simulink subsystem "ADIS16460"  (R2021a)
settings: Solver=VariableStepAuto  StartTime=0.0  StopTime=10.0  RelTol=1e-3
undefined symbols (not defined in the file): acc, gyro, max_ref_temp, misalign
libraries: simulink x8, dspsrcs4 x6, dspmtrx3 x2
settings Model: Creator=jmher  LastModifiedBy=Laura

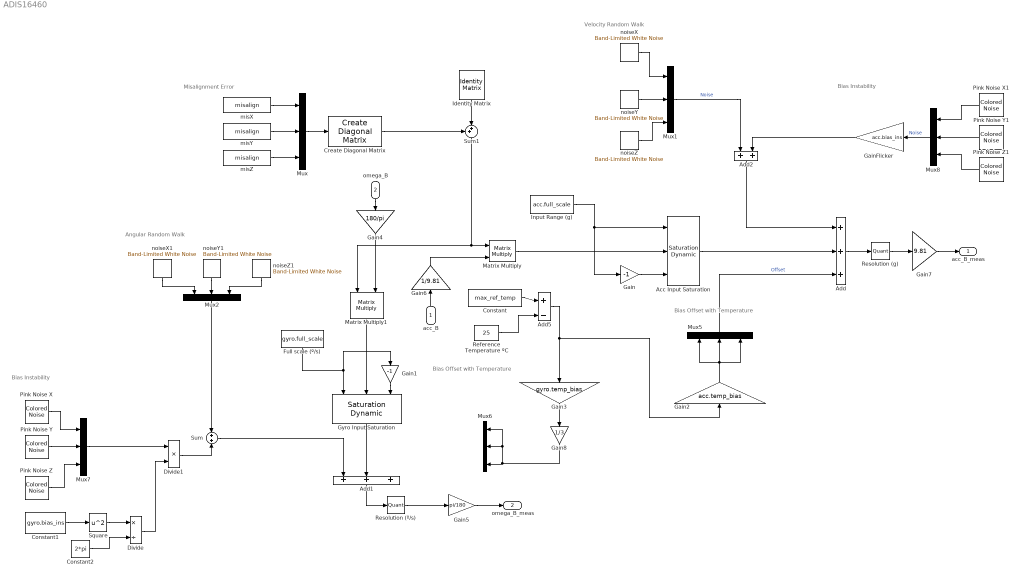
== system ADIS16460 ==
  note: Velocity Random Walk
  note: Bias Offset with Temperature
  note: Misalignment Error
  note: Bias Offset with Temperature
  note: Bias Instability
  note: Angular Random Walk
  note: Bias Instability
  acc_B : Inport  PortDimensions=3
  omega_B : Inport  Port=2  PortDimensions=3
  Acc Input Saturation : simulink/Discontinuities/Saturation Dynamic  OutMin=[]  OutMax=[]  OutDataTypeStr=Inherit: Same as second input  OutDataType=fixdt(1, 16)  OutScaling=2^-10  DoSatur=off
  Add : Sum  Inputs=+|+|+
  Add1 : Sum  Inputs=+|+|+
  Add2 : Sum  Inputs=+|+
  Add5 : Sum  Inputs=+|-
  Constant : Constant  Value=max_ref_temp
  Constant1 : Constant  Value=gyro.bias_ins
  Constant2 : Constant  Value=2*pi
  Create Diagonal Matrix : dspmtrx3/Create Diagonal Matrix
      settings: SourceProductBaseCode=DS
  Divide : Product  Inputs=*/
  Divide1 : Product  Inputs=**
  Full scale (º/s) : Constant  Value=gyro.full_scale
  Gain : Gain  Gain=-1
  Gain1 : Gain  Gain=-1
  Gain2 : Gain  Gain=acc.temp_bias
  Gain3 : Gain  Gain=gyro.temp_bias
  Gain4 : Gain  Gain=180/pi
  Gain5 : Gain  Gain=pi/180
  Gain6 : Gain  Gain=1/9.81
  Gain7 : Gain  Gain=9.81
  Gain8 : Gain  Gain=1/3
  GainFlicker : Gain  Gain=acc.bias_ins
  Gyro Input Saturation : simulink/Discontinuities/Saturation Dynamic  OutMin=[]  OutMax=[]  OutDataTypeStr=Inherit: Same as second input  OutDataType=fixdt(1, 16)  OutScaling=2^-10  DoSatur=off
  Identity Matrix : dspmtrx3/Identity Matrix  Inherit=off  N=3  Ts=1  dataType=double  isSigned=on  wordLen=16  udDataType=sfix(16)  fracBitsMode=Best precision  numFracBits=15  OutDataTypeStr=double  LastOutDataTypeStr=double
  Input Range (g) : Constant  Value=acc.full_scale
  Matrix Multiply : Product  Multiplication=Matrix(*)
  Matrix Multiply1 : Product  Multiplication=Matrix(*)
  Mux{,1..2,5..8} (7 alike) : Mux  Inputs=3
  Pink Noise X : dspsrcs4/Colored Noise  Color=pink  InverseFrequencyPower=biasAcc  BoundedOutput=off  NumChannels=1  OutputDataType=double  SamplesPerFrame=1  SampleTime=1/40  RandomStream=mt19937ar with seed  Seed=12237  SimulateUsing=Interpreted execution
      settings: SourceProductBaseCode=DS
  Pink Noise X1 : dspsrcs4/Colored Noise  Color=pink  InverseFrequencyPower=biasAcc  BoundedOutput=off  NumChannels=1  OutputDataType=double  SamplesPerFrame=1  SampleTime=1/40  RandomStream=mt19937ar with seed  Seed=6237342  SimulateUsing=Interpreted execution
      settings: SourceProductBaseCode=DS
  Pink Noise Y : dspsrcs4/Colored Noise  Color=pink  InverseFrequencyPower=biasAcc  BoundedOutput=off  NumChannels=1  OutputDataType=double  SamplesPerFrame=1  SampleTime=1/40  RandomStream=mt19937ar with seed  Seed=76372  SimulateUsing=Interpreted execution
      settings: SourceProductBaseCode=DS
  Pink Noise Y1 : dspsrcs4/Colored Noise  Color=pink  InverseFrequencyPower=biasAcc  BoundedOutput=off  NumChannels=1  OutputDataType=double  SamplesPerFrame=1  SampleTime=1/40  RandomStream=mt19937ar with seed  Seed=225421  SimulateUsing=Interpreted execution
      settings: SourceProductBaseCode=DS
  Pink Noise Z : dspsrcs4/Colored Noise  Color=pink  InverseFrequencyPower=biasAcc  BoundedOutput=off  NumChannels=1  OutputDataType=double  SamplesPerFrame=1  SampleTime=1/40  RandomStream=mt19937ar with seed  Seed=3755  SimulateUsing=Interpreted execution
      settings: SourceProductBaseCode=DS
  Pink Noise Z1 : dspsrcs4/Colored Noise  Color=pink  InverseFrequencyPower=biasAcc  BoundedOutput=off  NumChannels=1  OutputDataType=double  SamplesPerFrame=1  SampleTime=1/40  RandomStream=mt19937ar with seed  Seed=345617  SimulateUsing=Interpreted execution
      settings: SourceProductBaseCode=DS
  Reference Temperature ºC : Constant  Value=25
  Resolution (g) : Quantizer  QuantizationInterval=acc.quantization  LinearizeAsGain=off
  Resolution (º/s) : Quantizer  QuantizationInterval=gyro.quantization  LinearizeAsGain=off
  Square : Math  Operator=square  SaturateOnIntegerOverflow=on
  Sum : Sum
  Sum1 : Sum  Inputs=++|
  misX : Constant  Value=misalign
  misY : Constant  Value=misalign
  misZ : Constant  Value=misalign
  noiseX : simulink/Sources/Band-Limited White Noise  Cov=acc.power_noise(1)  Ts=1/40  seed=[32323556]
  noiseX1 : simulink/Sources/Band-Limited White Noise  Cov=gyro.power_noise(1)  Ts=1/40  seed=[3256]
  noiseY : simulink/Sources/Band-Limited White Noise  Cov=acc.power_noise(2)  Ts=1/40  seed=[238641]
  noiseY1 : simulink/Sources/Band-Limited White Noise  Cov=gyro.power_noise(2)  Ts=1/40  seed=[567380]
  noiseZ : simulink/Sources/Band-Limited White Noise  Cov=acc.power_noise(3)  Ts=1/40  seed=[23341231]
  noiseZ1 : simulink/Sources/Band-Limited White Noise  Cov=gyro.power_noise(3)  Ts=1/40  seed=[234234111]
  acc_B_meas : Outport  SampleTime=1/10
  omega_B_meas : Outport  Port=2  SampleTime=1/10
  wires:
  Pink Noise Z1/1 -> Mux8/3
  Gain6/1 -> Matrix Multiply/2
  Mux1/1 -> Add2/1  "Noise"
  noiseZ/1 -> Mux1/3
  Add/1 -> Resolution (g)/1
  Mux5/1 -> Add/3  "Offset"
  Identity Matrix/1 -> Sum1/2
  misZ/1 -> Mux/3
  Add5/1 -> Gain3/1, Gain2/1
  Mux/1 -> Create Diagonal Matrix/1
  Gain4/1 -> Matrix Multiply1/2
  Gain2/1 -> Mux5/1, Mux5/3, Mux5/2
  noiseZ1/1 -> Mux2/3
  Gain7/1 -> acc_B_meas/1
  omega_B/1 -> Gain4/1
  Pink Noise X1/1 -> Mux8/1
  noiseY/1 -> Mux1/2
  noiseX/1 -> Mux1/1
  Pink Noise X/1 -> Mux7/1
  Divide/1 -> Divide1/2
  Gain/1 -> Acc Input Saturation/3
  Gyro Input Saturation/1 -> Add1/2
  Resolution (º/s)/1 -> Gain5/1
  Acc Input Saturation/1 -> Add/2
  noiseY1/1 -> Mux2/2
  Matrix Multiply1/1 -> Gyro Input Saturation/2
  acc_B/1 -> Gain6/1
  Resolution (g)/1 -> Gain7/1
  Mux8/1 -> GainFlicker/1  "Noise"
  Mux7/1 -> Divide1/1
  Pink Noise Y/1 -> Mux7/2
  Pink Noise Z/1 -> Mux7/3
  Pink Noise Y1/1 -> Mux8/2
  Constant1/1 -> Square/1
  Constant2/1 -> Divide/2
  Mux2/1 -> Sum/1
  GainFlicker/1 -> Add2/2
  Divide1/1 -> Sum/2
  Full scale (º/s)/1 -> Gyro Input Saturation/1, Gain1/1
  Add2/1 -> Add/1
  Gain5/1 -> omega_B_meas/1
  noiseX1/1 -> Mux2/1
  Matrix Multiply/1 -> Acc Input Saturation/2
  misX/1 -> Mux/1
  misY/1 -> Mux/2
  Input Range (g)/1 -> Acc Input Saturation/1, Gain/1
  Square/1 -> Divide/1
  Gain1/1 -> Gyro Input Saturation/3
  Add1/1 -> Resolution (º/s)/1
  Constant/1 -> Add5/1
  Gain8/1 -> Mux6/3, Mux6/2, Mux6/1
  Gain3/1 -> Gain8/1
  Reference Temperature ºC/1 -> Add5/2
  Sum/1 -> Add1/1
  Create Diagonal Matrix/1 -> Sum1/1
  Sum1/1 -> Matrix Multiply1/1, Matrix Multiply/1
